simulink model "SIMULAZIONE_ECCESSO_PRODUZIONE"  (R2024a)
settings: Solver=VariableStepAuto  StartTime=0.0  StopTime=1800  RelTol=1e-3
undefined symbols (not defined in the file): cp, pitch, TSR
libraries: simulink x3, spsDCMachineLib x1, spsVoltageMeasurementLib x1, sps_lib x1
settings Model: Creator=emanuele  LastModifiedBy=emanuele

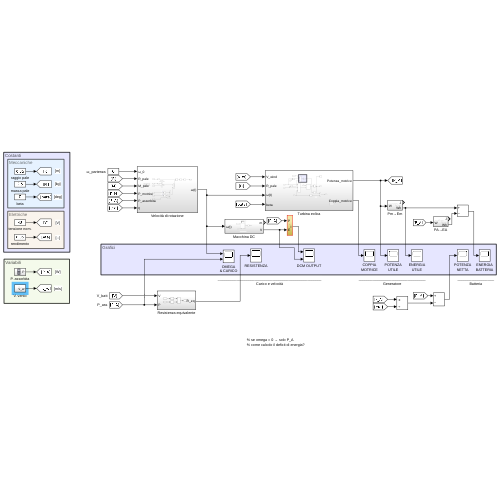
[thumbnail: Simulink's stored preview of the top-level diagram]
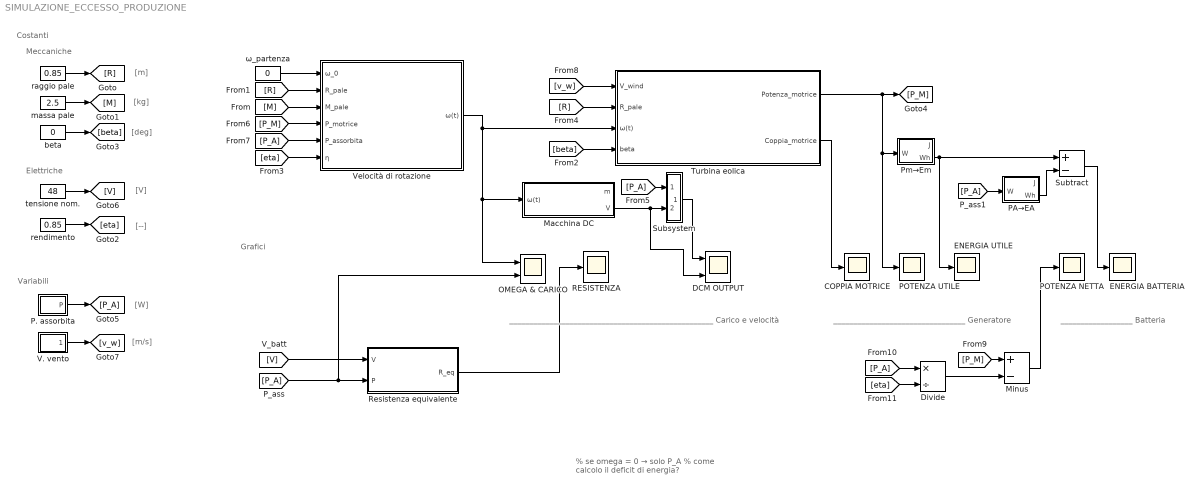
== system SIMULAZIONE_ECCESSO_PRODUZIONE ==
  note: ___________________________________________________
      | Carico e velocità
  note: % se omega = 0 → solo P_A
      | % come calcolo il deficit di energia?
  note: Elettriche
  note: Meccaniche
  note: Grafici
  note: Variabili
  note: [m]
  note: Costanti
  note: [kg]
  note: [deg]
  note: [--]
  note: [W]
  note: [V]
  note: [m/s]
  note: _________________________________
      | Generatore
  note: __________________
      | Batteria
  COPPIA MOTRICE : Scope
  DCM OUTPUT : Scope  NumInputPorts=2
  Divide : Product  Inputs=*/
  ENERGIA BATTERIA : Scope
  ENERGIA UTILE : Scope
  Macchina DC : Subsystem
  Minus : Sum  Inputs=+-
  OMEGA & CARICO : Scope  NumInputPorts=2
  P. assorbita : Subsystem
  PA→EA : Subsystem
  POTENZA NETTA : Scope
  POTENZA UTILE : Scope
  Pm→Em : Subsystem
  RESISTENZA : Scope
  Resistenza equivalente : Subsystem
  Subsystem : Subsystem
  Subtract : Sum  Inputs=+-
  Turbina eolica : Subsystem
  V. vento : Subsystem
  Velocità di rotazione : Subsystem
  beta : Constant  Value=0
  massa pale : Constant  Value=2.5
  raggio pale : Constant  Value=0.85
  rendimento : Constant  Value=0.85
  tensione nom. : Constant  Value=48
  ω_partenza : Constant  Value=0
  wires:
  ω_partenza/1 -> Velocità di rotazione/1(ω_0)
  Velocità di rotazione/1(ω(t)) -> Turbina eolica/3(ω(t)), Macchina DC/1(ω(t)), OMEGA & CARICO/1
  raggio pale/1 -> [R]
  massa pale/1 -> [M]
  beta/1 -> [beta]
  rendimento/1 -> [eta]
  [R] -> Velocità di rotazione/2(R_pale)
  [M] -> Velocità di rotazione/3(M_pale)
  [beta] -> Turbina eolica/4(beta)
  [eta] -> Velocità di rotazione/6(η)
  [R] -> Turbina eolica/2(R_pale)
  Turbina eolica/1(Potenza_motrice) -> [P_M], Pm→Em/1(W), POTENZA UTILE/1
  [P_M] -> Velocità di rotazione/4(P_motrice)
  Turbina eolica/2(Coppia_motrice) -> COPPIA MOTRICE/1
  [P_A] -> Velocità di rotazione/5(P_assorbita)
  P. assorbita/1(P) -> [P_A]
  tensione nom./1 -> [V]
  [P_A] -> OMEGA & CARICO/2, Resistenza equivalente/2(P)
  [V] -> Resistenza equivalente/1(V)
  Resistenza equivalente/1(R_eq) -> RESISTENZA/1
  [P_A] -> PA→EA/1(W)
  Pm→Em/2(Wh) -> ENERGIA UTILE/1, Subtract/1
  Subtract/1 -> ENERGIA BATTERIA/1
  PA→EA/2(Wh) -> Subtract/2
  Macchina DC/2(V) -> Subsystem/2(E), DCM OUTPUT/2
  [P_A] -> Subsystem/1(P)
  Subsystem/1(I) -> DCM OUTPUT/1
  [v_w] -> Turbina eolica/1(V_wind)
  [P_M] -> Minus/1
  Minus/1 -> POTENZA NETTA/1
  [eta] -> Divide/2
  [P_A] -> Divide/1
  Divide/1 -> Minus/2
  V. vento/1(v_w) -> [v_w]

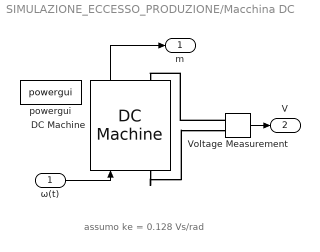
== system SIMULAZIONE_ECCESSO_PRODUZIONE/Macchina DC ==
  note: assumo ke = 0.128 Vs/rad
  ω(t) : Inport
  DC Machine : spsDCMachineLib/DC Machine  PresetModel=No  MechanicalLoad=Speed w  FieldType=Permanent magnet  ShowDetailedParameters=on  MeasurementBus=off  RLa="[ 0.6  0.012]"  RLf="[ 240  120]"  Laf=1.8  MachineConstant=Back-emf constant (V/rpm)  Ke=0.05  Kt=1.8  J=1  Bm=0  Tf=0  w0=1  Ifinit=1  TsPowergui=0  TsBlock=-1
  Voltage Measurement : spsVoltageMeasurementLib/Voltage Measurement  PhasorSimulation=off  OutputType=Complex  PSBequivalent=0
  powergui : sps_lib/powergui  Priority=1  SimulationMode=Continuous  SampleTime=50e-6  frequency=60  Iterations=50  frequencyindice=0  Pbase=100e6  ErrMax=1e-4  UnitsV=kV  UnitsW=MW  buscounter=0  FunctionMessages=off  echomessages=off  EnableUseOfTLC=off  CurrentSourceSwitches=off  DisableSnubberDevices=off  DisableRonSwitches=off  DisableVfSwitches=off  DisplayEquations=off  AutomaticDiscreteSolvers=off  SolverType=Tustin/Backward Euler (TBE)  Interpol=off  ExternalGateDelay=off  methode=off  Ts=100  x0status=blocks  SPID=on  SwTol=0  HookPort=off  NonlinearTolerance=1e-4  nMaxIteration=100  ContinueOnMaxIteration=off  RestoreLinks=warning  ResistiveCurrentMeasurement=off  Frange=[0:2:500]  Ylog=off  Xlog=on  ShowGrid=off  save=off  variable=ZData  structure=0  ZoomFFT=off  StartTime=0.0  cycles=1  DisplayStyle=1  fundamental=60  FreqAxis=off  MaxFrequency=1000  frequencyindicesteady=1  RmsSteady=1  display=off
  m : Outport
  V : Outport  Port=2  Unit=V
  wires:
  ω(t)/1 -> DC Machine/1
  DC Machine/1 -> m/1
  Voltage Measurement/1 -> V/1
  connections:
  Voltage Measurement/LConn2 -- DC Machine/RConn1
  DC Machine/LConn1 -- Voltage Measurement/LConn1

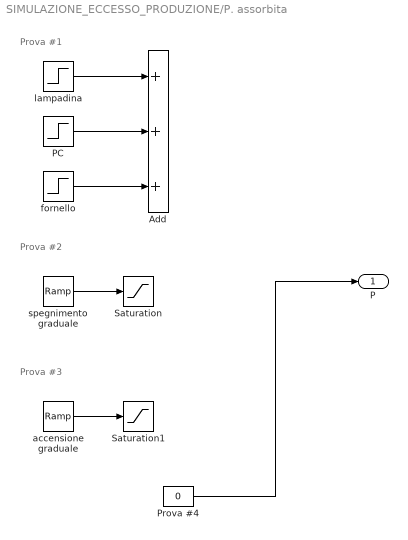
== system SIMULAZIONE_ECCESSO_PRODUZIONE/P. assorbita ==
  note: Prova #1
  note: Prova #2
  note: Prova #3
  Add : Sum  Inputs=+++
  PC : Step  Time=1200  After=90  SampleTime=0
  Prova #4 : Constant  Value=0
  Saturation : Saturate  UpperLimit=1000  LowerLimit=0
  Saturation1 : Saturate  UpperLimit=200  LowerLimit=0
  accensione graduale : simulink/Sources/Ramp  slope=2  start=900  InitialOutput=0
  fornello : Step  Time=1500  After=900  SampleTime=0
  lampadina : Step  Time=900  After=10  SampleTime=0
  spegnimento graduale : simulink/Sources/Ramp  slope=-10  start=900  InitialOutput=1000
  P : Outport
  wires:
  lampadina/1 -> Add/1
  PC/1 -> Add/2
  fornello/1 -> Add/3
  spegnimento graduale/1 -> Saturation/1
  accensione graduale/1 -> Saturation1/1
  Prova #4/1 -> P/1

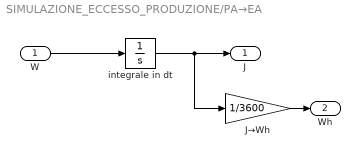
== system SIMULAZIONE_ECCESSO_PRODUZIONE/PA→EA ==
  W : Inport
  J→Wh : Gain  Gain=1/3600
  integrale in dt : Integrator
  J : Outport  Unit=J
  Wh : Outport  Port=2  Unit=W*h
  wires:
  W/1 -> integrale in dt/1
  J→Wh/1 -> Wh/1
  integrale in dt/1 -> J→Wh/1, J/1

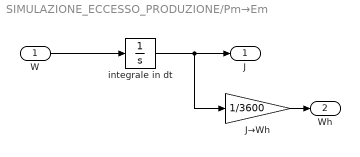
== system SIMULAZIONE_ECCESSO_PRODUZIONE/Pm→Em ==
  W : Inport
  J→Wh : Gain  Gain=1/3600
  integrale in dt : Integrator
  J : Outport  Unit=J
  Wh : Outport  Port=2  Unit=W*h
  wires:
  integrale in dt/1 -> J/1, J→Wh/1
  J→Wh/1 -> Wh/1
  W/1 -> integrale in dt/1

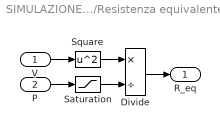
== system SIMULAZIONE_ECCESSO_PRODUZIONE/Resistenza equivalente ==
  V : Inport  Unit=V
  P : Inport  Port=2
  Divide : Product  Inputs=*/
  Saturation : Saturate  UpperLimit=10e4  LowerLimit=10e-1
  Square : Math  Operator=square
  R_eq : Outport  Unit=Ω
  wires:
  Divide/1 -> R_eq/1
  V/1 -> Square/1
  Square/1 -> Divide/1
  P/1 -> Saturation/1
  Saturation/1 -> Divide/2

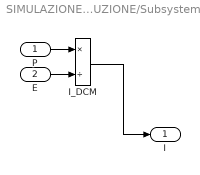
== system SIMULAZIONE_ECCESSO_PRODUZIONE/Subsystem ==
  P : Inport  Unit=W
  E : Inport  Port=2  Unit=V
  I_DCM : Product  Inputs=*/
  I : Outport  Unit=A
  wires:
  P/1 -> I_DCM/1
  E/1 -> I_DCM/2
  I_DCM/1 -> I/1

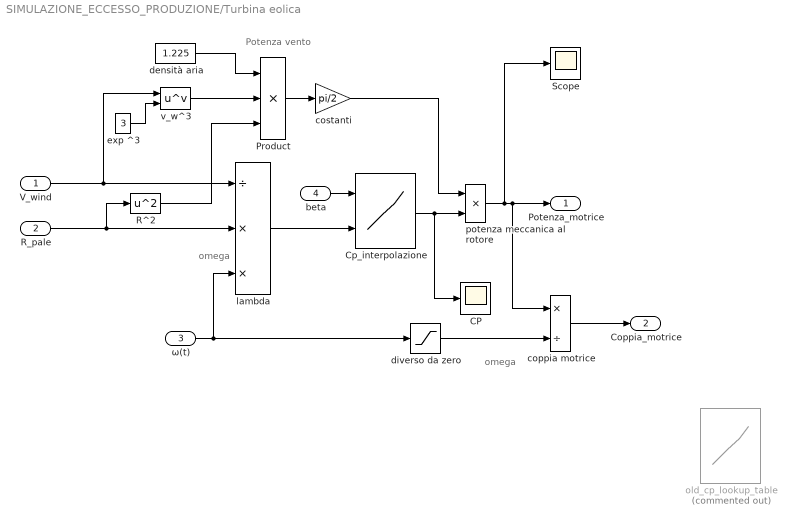
== system SIMULAZIONE_ECCESSO_PRODUZIONE/Turbina eolica ==
  note: Potenza vento
  note: omega
  note: omega
  V_wind : Inport  Unit=m/s
  R_pale : Inport  Port=2  Unit=m
  ω(t) : Inport  Port=3
  beta : Inport  Port=4  Unit=deg
  CP : Scope
  Cp_interpolazione : Lookup_n-D  BreakpointsForDimension1=pitch  BreakpointsForDimension2=TSR  Table=cp  InterpMethod=Cubic spline  InternalRulePriority=Speed  RndMeth=Simplest
      settings: InputPortMap=u0,u1
  Product : Product  Inputs=***
  R^2 : Math  Operator=square
  Scope : Scope
  coppia motrice : Product  Inputs=*/
  costanti : Gain  Gain=pi/2
  densità aria : Constant  Value=1.225
  diverso da zero : Saturate  UpperLimit=10e3  LowerLimit=0.1
  exp ^3 : Constant  Value=3
  lambda : Product  Inputs=/**
  old_cp_lookup_table : Lookup_n-D  Commented=on  BreakpointsForDimension1=[0, 3, 5, 10, 20, 90]  BreakpointsForDimension2=[0, 2, 4, 6, 8, 10, 12, 14, 15]  Table=[0.0010, 0.0161, 0.1446, 0.3865, 0.5009, 0.4404, 0.2545, 0.0002, -0.1384; 0.0016, 0.0173, 0.1079, 0.2676, 0.3779, 0.4111, 0.3838, 0.3176, 0.2753; 0.0027, 0.0197, 0.1151, 0.2606, 0.3469, 0.3558, 0.3069, 0.2222, 0.1718; 0.0054, 0.0283, 0.1315, 0.2364, 0.2589, 0.2022, 0.0929, -0.0455, -0.1204; 0.0109, 0.0536, 0.1320, 0.1256, 0.0120, -0.1752, -0.4017, -0.6435, -0.7655; -0.01 * ones(1, 9)]  InterpMethod=Linear Lagrange  InternalRulePriority=Speed  RndMeth=Simplest
      settings: InputPortMap=u0,u1
  potenza meccanica al rotore : Product
  v_w^3 : Math  Operator=pow
  Potenza_motrice : Outport  Unit=W
  Coppia_motrice : Outport  Port=2  Unit=N*m
  wires:
  potenza meccanica al rotore/1 -> Scope/1, Potenza_motrice/1, coppia motrice/1
  R_pale/1 -> lambda/2, R^2/1
  V_wind/1 -> lambda/1, v_w^3/1
  densità aria/1 -> Product/1
  v_w^3/1 -> Product/2
  R^2/1 -> Product/3
  Product/1 -> costanti/1
  Cp_interpolazione/1 -> CP/1, potenza meccanica al rotore/2
  beta/1 -> Cp_interpolazione/1
  lambda/1 -> Cp_interpolazione/2
  ω(t)/1 -> diverso da zero/1, lambda/3
  diverso da zero/1 -> coppia motrice/2
  coppia motrice/1 -> Coppia_motrice/1
  costanti/1 -> potenza meccanica al rotore/1
  exp ^3/1 -> v_w^3/2

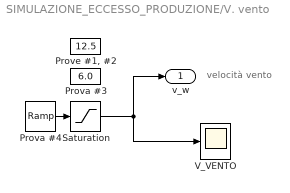
== system SIMULAZIONE_ECCESSO_PRODUZIONE/V. vento ==
  note: velocità vento
  Prova #3 : Constant  Value=6.0
  Prova #4 : simulink/Sources/Ramp  slope=0.1  start=900  InitialOutput=2
  "Prove #1, #2" : Constant  Value=12.5
  Saturation : Saturate  UpperLimit=20  LowerLimit=10e-2
  V_VENTO : Scope
  v_w : Outport
  wires:
  Prova #4/1 -> Saturation/1
  Saturation/1 -> v_w/1, V_VENTO/1

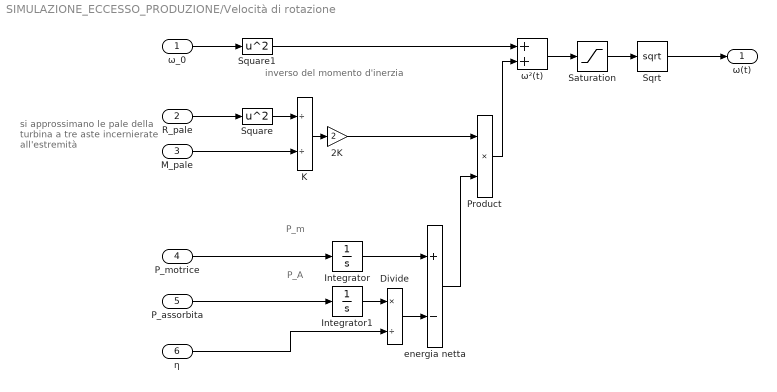
== system SIMULAZIONE_ECCESSO_PRODUZIONE/Velocità di rotazione ==
  note: si approssimano le pale
      | della turbina a tre aste
      | incernierate all'estremità
  note: inverso del
      | momento d'inerzia
  note: P_A
  note: P_m
  ω_0 : Inport  Unit=rad/s
  R_pale : Inport  Port=2  Unit=m
  M_pale : Inport  Port=3  Unit=kg
  P_motrice : Inport  Port=4  Unit=W
  P_assorbita : Inport  Port=5  Unit=W
  η : Inport  Port=6  Unit=1
  2K : Gain  Gain=2
  Divide : Product  Inputs=*/
  Integrator : Integrator
  Integrator1 : Integrator
  K : Product  Inputs=//
  Product : Product
  Saturation : Saturate  UpperLimit=10e6  LowerLimit=0
  Sqrt : Sqrt
  Square : Math  Operator=square
  Square1 : Math  Operator=square
  energia netta : Sum  Inputs=+-
  ω²(t) : Sum
  ω(t) : Outport  Unit=rad/s
  wires:
  M_pale/1 -> K/2
  K/1 -> 2K/1
  Sqrt/1 -> ω(t)/1
  energia netta/1 -> Product/2
  Integrator/1 -> energia netta/1
  R_pale/1 -> Square/1
  P_assorbita/1 -> Integrator1/1
  Integrator1/1 -> Divide/1
  Product/1 -> ω²(t)/2
  Square/1 -> K/1
  P_motrice/1 -> Integrator/1
  Square1/1 -> ω²(t)/1
  ω_0/1 -> Square1/1
  ω²(t)/1 -> Saturation/1
  2K/1 -> Product/1
  Divide/1 -> energia netta/2
  η/1 -> Divide/2
  Saturation/1 -> Sqrt/1
